simulink model "BatterySOCEstimation_by_me_3"  (R2024b)
settings: Solver=VariableStepAuto  StartTime=0.0  StopTime=1500  FixedStep=Ts  RelTol=1e-3  EnableMultiTasking=on
PreLoadFcn:
  | BatterySOCEstimationData;
libraries: fl_lib x8, nesl_utility x5, simulink x3, batteryecm_lib x1, BatteryEstimators x1
CloseFcn:
  | try
  |     close(h1_BatterySOCEstimation)
  | catch
  | end
  | 
  | clear h1_BatterySOCEstimation
  | 
  | clear BatterySOCEstimationSimlog
  | clear BatterySOCEstimationLogsout
  | 
  | clear AH SOC_vec T_vec R0_mat R1_mat tau1_mat
  | clear V0_mat Q R P0 initialSOC SOC0 Ts
  | clear cell_area h_conv thermal_mass
Description:
  | Battery State-of-Charge Estimation
settings Model: Creator=The MathWorks, Inc.  LastModifiedBy=nikhi
settings SolverCC: AlgebraicLoopSolver=TrustRegion  AutoInsertRateTranBlk=on  MaxZcPerStep=1
settings DataIOCC: MaxDataPoints=370000  ReturnWorkspaceOutputs=off  SignalLoggingName=BatterySOCEstimationLogsout
settings OptimizationCC: ReuseModelBlockBuffer=off  LifeSpan=inf
settings DebuggingCC: UnconnectedInputMsg=warning  UnconnectedOutputMsg=warning  UnconnectedLineMsg=warning  SFUnexpectedBacktrackingDiag=warning  SFNoUnconditionalDefaultTransitionDiag=warning  SFExecutionAtInitializationDiag=none  ArithmeticOperatorsInVariantConditions=warning
settings ModelReferenceCC: EnableRefExpFcnMdlSchedulingChecks=on
settings SFSimCC: SimUseLocalCustomCode=off  CustomCodeUndefinedFunction=UseInterfaceOnly
settings RTWCC: RTWUseLocalCustomCode=off  GPUComputeCapability=3.5  DLArmComputeVersion=19.05
settings CodeAppCC: StateflowObjectComments=on
settings GRTTargetCC: TargetLangStandard=C89/C90 (ANSI)
settings ConfigComp: CovMetricSettings=dw  CovSaveCumulativeToWorkspaceVar=on  CovSaveSingleToWorkspaceVar=on  CovExternalEMLEnable=off
settings SimscapeCC: SimscapeLogType=all  SimscapeLogSimulationStatistics=on  SimscapeLogName=BatterySOCEstimationSimlog  SimscapeLogLimitData=off  SimscapeLogDataHistory=370000

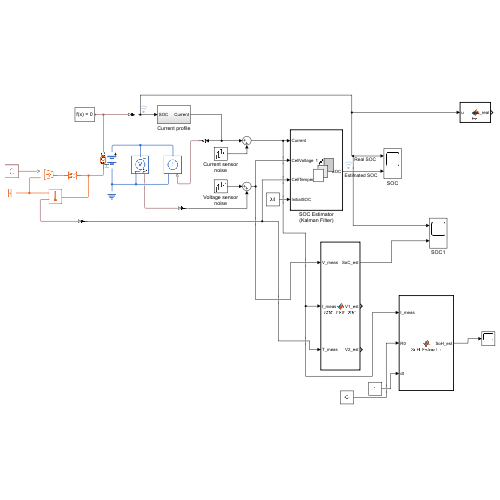
[thumbnail: Simulink's stored preview of the top-level diagram]
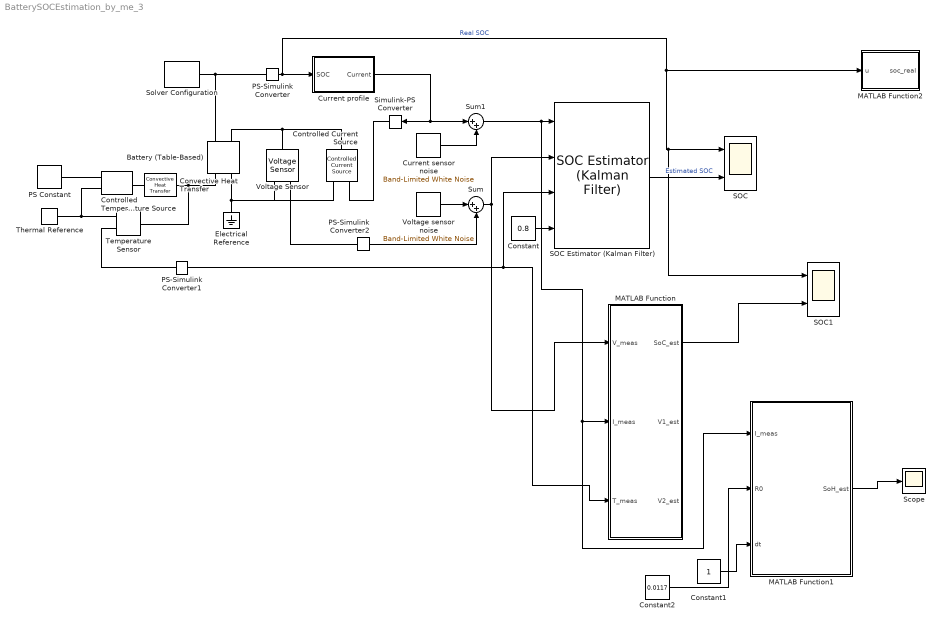
== system BatterySOCEstimation_by_me_3 ==
  Battery (Table-Based) : batteryecm_lib/Battery (Table-Based)  SOC_vec=[0 0.1 0.25 0.5 0.75 0.9 1]  T_dependence=simscape.enum.tablebattery.temperature_dependence.yes  prm_dir=simscape.enum.tablebattery.prm_dir.noCurrentDirectionality  T_vec=[278,293,313] K  V0_mat=[3.49 3.5 3.51;3.55 3.57 3.56;3.62 3.63 3.64;3.71 3.71 3.72;3.91 3.93 3.94;4.07 4.08 4.08;4.19 4.19 4.19] V  V0_vec=[3.5057, 3.566, 3.6337, 3.7127, 3.9259, 4.0777, 4.1928] V  V_range=[0, inf] V  R0_mat=[0.0117 0.0085 0.009;0.011 0.0085 0.009;0.0114 0.0087 0.0092;0.0107 0.0082 0.0088;0.0107 0.0083 0.0091;0.0113 0.0085 0.0089;0.0116 0.0085 0.0089] Ohm  R0_vec=[.0085, .0085, .0087, .0082, .0083, .0085, .0085] Ohm  R0_dis_mat=[.0117, .0085, .009; .011, .0085, .009; .0114, .0087, .0092; .0107, .0082, .0088; .0107, .0083, .0091; .0113, .0085, .0089; .0116, .0085, .0089] Ohm  R0_dis_vec=[.0085, .0085, .0087, .0082, .0083, .0085, .0085] Ohm  R0_ch_mat=[.0117, .0085, .009; .011, .0085, .009; .0114, .0087, .0092; .0107, .0082, .0088; .0107, .0083, .0091; .0113, .0085, .0089; .0116, .0085, .0089] Ohm  R0_ch_vec=[.0085, .0085, .0087, .0082, .0083, .0085, .0085] Ohm  AH=10 A*hr  prm_leak=simscape.enum.tablebattery.prm_leak.disabled  Rleak_vec=[8000, 7000, 6000] Ohm  Rleak=7e3 Ohm  extrapolation_option=simscape.enum.extrapolation.nearest  SOC_port=simscape.enum.tablebattery.enable.yes  prm_dyn=simscape.enum.tablebattery.prm_dyn.rc1  R1_mat=[0.0109 0.0029 0.0013;0.0069 0.0024 0.0012;0.0047 0.0026 0.0013;0.0034 0.0016 0.001;0.0033 0.0023 0.0014;0.0033 0.0018 0.0011;0.0028 0.0017 0.0011] Ohm  R1_vec=[.0029, .0024, .0026, .0016, .0023, .0018, .0017] Ohm  tau1_mat=[20 36 39;31 45 39;109 105 61;36 29 26;59 77 67;40 33 29;25 39 33] s  tau1_vec=[36, 45, 105, 29, 77, 33, 39] s  R2_mat=[.0109, .0029, .0013; .0069, .0024, .0012; .0047, .0026, .0013; .0034, .0016, .001; .0033, .0023, .0014; .0033, .0018, .0011; .0028, .0017, .0011] Ohm  R2_vec=[.0029, .0024, .0026, .0016, .0023, .0018, .0017] Ohm  tau2_mat=[20, 36, 39; 31, 45, 39; 109, 105, 61; 36, 29, 26; 59, 77, 67; 40, 33, 29; 25, 39, 33] s  tau2_vec=[36, 45, 105, 29, 77, 33, 39] s  R3_mat=[.0109, .0029, .0013; .0069, .0024, .0012; .0047, .0026, .0013; .0034, .0016, .001; .0033, .0023, .0014; .0033, .0018, .0011; .0028, .0017, .0011] Ohm  R3_vec=[.0029, .0024, .0026, .0016, .0023, .0018, .0017] Ohm  tau3_mat=[20, 36, 39; 31, 45, 39; 109, 105, 61; 36, 29, 26; 59, 77, 67; 40, 33, 29; 25, 39, 33] s  tau3_vec=[36, 45, 105, 29, 77, 33, 39] s  R4_mat=[.0109, .0029, .0013; .0069, .0024, .0012; .0047, .0026, .0013; .0034, .0016, .001; .0033, .0023, .0014; .0033, .0018, .0011; .0028, .0017, .0011] Ohm  R4_vec=[.0029, .0024, .0026, .0016, .0023, .0018, .0017] Ohm  tau4_mat=[20, 36, 39; 31, 45, 39; 109, 105, 61; 36, 29, 26; 59, 77, 67; 40, 33, 29; 25, 39, 33] s  tau4_vec=[36, 45, 105, 29, 77, 33, 39] s  R5_mat=[.0109, .0029, .0013; .0069, .0024, .0012; .0047, .0026, .0013; .0034, .0016, .001; .0033, .0023, .0014; .0033, .0018, .0011; .0028, .0017, .0011] Ohm  R5_vec=[.0029, .0024, .0026, .0016, .0023, .0018, .0017] Ohm  tau5_mat=[20, 36, 39; 31, 45, 39; 109, 105, 61; 36, 29, 26; 59, 77, 67; 40, 33, 29; 25, 39, 33] s  tau5_vec=[36, 45, 105, 29, 77, 33, 39] s  prm_fade=simscape.enum.tablebattery.prm_fade.disabled  N0=10  dV0=0  dR0=500  dAH=0  dRleak=0  dR1=0  dR2=0  dR3=0  dR4=0  dR5=0  N0vec=[100, 200, 300]  Tfadevec=[298.15, 323.15] K  dV0vec=[0, 0, 0]  dR0vec=[0, 0, 0]  dAHvec=[0, 0, 0]  dRleakvec=[0, 0, 0]  dR1vec=[0, 0, 0]  dR2vec=[0, 0, 0]  dR3vec=[0, 0, 0]  dR4vec=[0, 0, 0]  dR5vec=[0, 0, 0]  dV0mat=[0, 0; 0, 0; 0, 0]  dR0mat=[0, 0; 0, 0; 0, 0]  dAHmat=[0, 0; 0, 0; 0, 0]  dRleakmat=[0, 0; 0, 0; 0, 0]  dR1mat=[0, 0; 0, 0; 0, 0]  dR2mat=[0, 0; 0, 0; 0, 0]  dR3mat=[0, 0; 0, 0; 0, 0]  dR4mat=[0, 0; 0, 0; 0, 0]  dR5mat=[0, 0; 0, 0; 0, 0]  prm_age_modeling=simscape.enum.tablebattery.prm_age_modeling.equation  storage_dt_age_vec=[0] d  storage_T_age_vec=[273] K  prm_age_OCV=simscape.enum.tablebattery.prm_age_OCV.OCV  OCV_age=0.9  SOC_age=0.6  prm_age_resistance=simscape.enum.tablebattery.prm_age.disabled  OCV_scaling_age_resistance=2.2134e6  OCV_offset_age_resistance=1.632e6  temp_exp_age_resistance=0.515833569 V  t_exp_age_resistance=0.75  T_age_vec_resistance=[273.15, 298.15, 323.15] K  dt_age_vec_resistance=[90, 180, 270, 360] d  dR0_age_vec=[0, 0, 0]  t_meas_dR0_age=100 d  dR0_age_mat=[0, 0, 0; 0, 0, 0; 0, 0, 0; 0, 0, 0]  prm_age_capacity=simscape.enum.tablebattery.prm_age.disabled  OCV_scaling_age_capacity=1.5097e07  OCV_offset_age_capacity=8.3625e06  temp_exp_age_capacity=0.6011 V  t_exp_age_capacity=0.75  T_age_vec_capacity=[273.15, 298.15, 323.15] K  dt_age_vec_capacity=[90, 180, 270, 360] d  dAH_age_vec=[0, 0, 0]  t_meas_dAH_age=100 d  dAH_age_mat=[0, 0, 0; 0, 0, 0; 0, 0, 0; 0, 0, 0]  thermal_port=simscape.enum.thermaleffects.model  temperature=298.15 K  thermal_mass=100 J/K  i_specify=off  i_priority=None  i=0 A  i_nominal_specify=off  i_nominal_value=1  i_nominal_unit=A  v_specify=off  v_priority=None  v=0 V  v_nominal_specify=off  v_nominal_value=1  v_nominal_unit=V  stateOfCharge_specify=on  stateOfCharge_priority=High  stateOfCharge=0.5  stateOfCharge_nominal_specify=off  stateOfCharge_nominal_value=1  stateOfCharge_nominal_unit=1  num_cycles_specify=off  num_cycles_priority=High  num_cycles=0  num_cycles_nominal_specify=off  num_cycles_nominal_value=1  num_cycles_nominal_unit=1  cell_temperature_specify=off  cell_temperature_priority=High  cell_temperature=293.15 K  cell_temperature_nominal_specify=off  cell_temperature_nominal_value=1  cell_temperature_nominal_unit=K
  Constant : Constant  Value=0.8
  Constant1 : Constant
  Constant2 : Constant  Value=0.0117
  Controlled Temperature Source : fl_lib/Thermal/Thermal Sources/Controlled Temperature Source
  Controlled Current Source : fl_lib/Electrical/Electrical Sources/Controlled Current Source
  Convective Heat Transfer : fl_lib/Thermal/Thermal Elements/Convective Heat Transfer  thermal_type=foundation.enum.constant_variable.constant  area=0.1019 m^2  heat_tr_coeff=5 W/(K*m^2)  min_heat_tr_coeff=1e-3 W/(K*m^2)  T_specify=off  T_priority=None  T=0 K  T_nominal_specify=off  T_nominal_value=1  T_nominal_unit=K  Q_specify=off  Q_priority=None  Q=0 W  Q_nominal_specify=off  Q_nominal_value=1  Q_nominal_unit=W
  Current profile : Subsystem
  Current sensor noise : simulink/Sources/Band-Limited White Noise  Cov=1e-2  Ts=1  seed=1234
  Electrical Reference : fl_lib/Electrical/Electrical Elements/Electrical Reference
  MATLAB Function : MATLAB Function  TreatAsAtomicUnit=on
  MATLAB Function1 : MATLAB Function  TreatAsAtomicUnit=on
  MATLAB Function2 : MATLAB Function  TreatAsAtomicUnit=on
  PS Constant : fl_lib/Physical Signals/Sources/PS Constant  constant=292.15 K
  PS-Simulink Converter : nesl_utility/PS-Simulink Converter  PhysicalDomain=network_engine_domain  SubClassName=ps_output  LeftPortType=input  RightPortType=output  PseudoPeriodic=off  Frequencies=[]  VectorFormat=inherit  Unit=inherit  AffineConversion=off
  PS-Simulink Converter1 : nesl_utility/PS-Simulink Converter  PhysicalDomain=network_engine_domain  SubClassName=ps_output  LeftPortType=input  RightPortType=output  PseudoPeriodic=off  Frequencies=[]  VectorFormat=inherit  Unit=inherit  AffineConversion=off
  PS-Simulink Converter2 : nesl_utility/PS-Simulink Converter  PhysicalDomain=network_engine_domain  SubClassName=ps_output  LeftPortType=input  RightPortType=output  PseudoPeriodic=off  Frequencies=[]  VectorFormat=inherit  Unit=inherit  AffineConversion=off
  SOC : Scope  NumInputPorts=2
  SOC Estimator (Kalman Filter) : BatteryEstimators/SOC Estimator (Kalman Filter)  CurrentInputPartition=off  filterType=Extended Kalman filter  alpha=1  beta=2  kappa=0  Q=[0.0001,0;0,0.0001]  Q_2RC=|  R=0.7  P0=[1e-05,0;0,1]  P0_2RC=[1e-5 0 0; 0 1 0;0 0 1]  Ts=1  chargeDynamics=One time-constant dynamics  SOC_vec=[0 0.1 0.25 0.5 0.75 0.9 1]  T_vec=[278,293,313]  R0_mat=[0.0117 0.0085 0.009;0.011 0.0085 0.009;0.0114 0.0087 0.0092;0.0107 0.0082 0.0088;0.0107 0.0083 0.0091;0.0113 0.0085 0.0089;0.0116 0.0085 0.0089]  R1_mat=[0.0109 0.0029 0.0013;0.0069 0.0024 0.0012;0.0047 0.0026 0.0013;0.0034 0.0016 0.001;0.0033 0.0023 0.0014;0.0033 0.0018 0.0011;0.0028 0.0017 0.0011]  tau1_mat=[20 36 39;31 45 39;109 105 61;36 29 26;59 77 67;40 33 29;25 39 33]  R2_mat=[.0109, .0029, .0013; .0069, .0024, .0012; .0047, .0026, .0013; .0034, .0016, .001; .0033, .0023, .0014; .0033, .0018, .0011; .0028, .0017, .0011]  tau2_mat=[20, 36, 39; 31, 45, 39; 109, 105, 61; 36, 29, 26; 59, 77, 67; 40, 33, 29; 25, 39, 33]  V0_mat=[3.49 3.5 3.51;3.55 3.57 3.56;3.62 3.63 3.64;3.71 3.71 3.72;3.91 3.93 3.94;4.07 4.08 4.08;4.19 4.19 4.19]  AH=10
      | [1e-6 0 0;
      | 0 1e-6 0; 0 0 1e-6]
  SOC1 : Scope  NumInputPorts=2
  Scope : Scope
  Simulink-PS Converter : nesl_utility/Simulink-PS Converter  PhysicalDomain=network_engine_domain  SubClassName=ps_input  LeftPortType=input  RightPortType=output  PseudoPeriodic=off  Frequencies=[]  NoiseDistribution=none  NoiseParameters=[]  Unit=1  AffineConversion=off  FilteringAndDerivatives=provide  SimscapeFilterOrder=1  InputFilterTimeConstant=0.001  UdotUserProvided=0
  Solver Configuration : nesl_utility/Solver Configuration  PhysicalDomain=network_engine_domain  SubClassName=solver  LeftPortType=input  RightPortType=generic  Tones=[]  Harmonics=[]  SimulateNoise=off  Profile=off  UseLocalSampling=off  EnableSwitchedLinearOptims=on  FrequencyDomain=off  UseCCode=off  RelTol=0.001  AbsTol=0.001  MinStep=1e-09  ToWorkspace=off  RevertToSquareIcSolve=off  NumHomotopyIterations=100  PhasorMode=off  PhasorModeNumHarmonics=1  ConsistencySolver=NEWTON_XTOL_AFTER_FTOL  IndexReductionMethod=DerivativeReplacement  DoDC=off  ResidualTolerance=1e-09  ConsistencyTolSource=GLOBAL  ConsistencyAbsTol=0.001  ConsistencyRelTol=0.001  ConsistencyTolFactor=0.001  UseLocalSolver=on  LocalSolverChoice=NE_BACKWARD_EULER_ADVANCER  ResolveIndetEquations=on  FunctionEvalNumThread=1  LocalSolverSampleTime=1  DoFixedCost=on  MaxNonlinIter=3  MaxModeIter=2  ComputeImpulses=off  ImpulseIterations=2  LinearAlgebra=auto  LinearAlgebraNumThread=0  EquationFormulation=NE_TIME_EF  DelaysMemoryBudget=1024  AutomaticFiltering=on  FilteringTimeConstant=0.001  PartitionStorageMethod=AS_NEEDED  PartitionMemoryBudget=1024  PartitionMethod=ROBUST  MultibodyUseLocalSolver=off  MultibodyLocalSolverChoice=ODE1  MultibodyLocalSolverSampleTime=0.001
  Sum : Sum  Inputs=|++
  Sum1 : Sum  Inputs=|++
  Temperature Sensor : fl_lib/Thermal/Thermal Sensors/Temperature Sensor  temperature_measure=foundation.enum.MeasurementReference.difference
  Thermal Reference : fl_lib/Thermal/Thermal Elements/Thermal Reference
  Voltage Sensor : fl_lib/Electrical/Electrical Sensors/Voltage Sensor
  Voltage sensor noise : simulink/Sources/Band-Limited White Noise  Cov=1e-2  Ts=1  seed=1234
  wires:
  PS-Simulink Converter2/1 -> Sum/2
  Current sensor noise/1 -> Sum1/2
  Constant/1 -> SOC Estimator (Kalman Filter)/4
  SOC Estimator (Kalman Filter)/1 -> SOC/2  "Estimated SOC"
  PS-Simulink Converter/1 -> MATLAB Function2/1(u), SOC1/1, SOC/1, Current profile/1(SOC)  "Real SOC"
  Voltage sensor noise/1 -> Sum/1
  Current profile/1(Current) -> Sum1/1, Simulink-PS Converter/1
  MATLAB Function/1(SoC_est) -> SOC1/2
  Sum/1 -> MATLAB Function/1(V_meas), SOC Estimator (Kalman Filter)/2
  Sum1/1 -> MATLAB Function1/1(I_meas), MATLAB Function/2(I_meas), SOC Estimator (Kalman Filter)/1
  PS-Simulink Converter1/1 -> MATLAB Function/3(T_meas), SOC Estimator (Kalman Filter)/3
  Constant1/1 -> MATLAB Function1/3(dt)
  Constant2/1 -> MATLAB Function1/2(R0)
  MATLAB Function1/1(SoH_est) -> Scope/1
  connections:
  PS-Simulink Converter/LConn1 -- Solver Configuration/RConn1 -- Battery (Table-Based)/LConn2
  Convective Heat Transfer/LConn1 -- Temperature Sensor/LConn1 -- Battery (Table-Based)/RConn2
  Controlled Temperature Source/LConn1 -- Convective Heat Transfer/RConn1
  Thermal Reference/LConn1 -- Controlled Temperature Source/RConn2 -- Temperature Sensor/RConn1
  PS-Simulink Converter1/LConn1 -- Temperature Sensor/RConn2
  Electrical Reference/LConn1 -- Voltage Sensor/RConn2 -- Controlled Current Source/RConn2 -- Battery (Table-Based)/RConn1
  Voltage Sensor/LConn1 -- Controlled Current Source/LConn1 -- Battery (Table-Based)/LConn1
  Simulink-PS Converter/RConn1 -- Controlled Current Source/RConn1
  Voltage Sensor/RConn1 -- PS-Simulink Converter2/LConn1
  PS Constant/RConn1 -- Controlled Temperature Source/RConn1

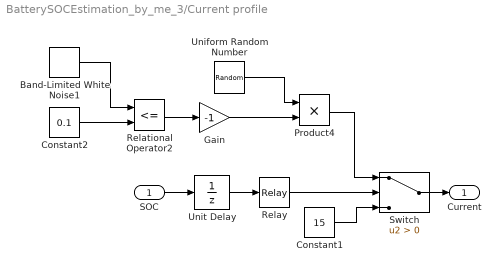
== system BatterySOCEstimation_by_me_3/Current profile ==
  SOC : Inport
  Band-Limited White Noise1 : simulink/Sources/Band-Limited White Noise  Cov=1  Ts=50  seed=[23341]
  Constant1 : Constant  Value=15
  Constant2 : Constant  Value=0.1
  Gain : Gain  Gain=-1
  Product4 : Product
  Relational Operator2 : RelationalOperator  Operator=<=  OutDataTypeStr=boolean  RndMeth=Simplest  InputSameDT=off
  Relay : Relay  OnSwitchValue=0.9  OffSwitchValue=0.3  OffOutputValue=-1
  Switch : Switch  Criteria=u2 > Threshold  SaturateOnIntegerOverflow=off  InputSameDT=off
  Uniform Random Number : UniformRandomNumber  Minimum=5  Maximum=55  SampleTime=100
  Unit Delay : UnitDelay  HasFrameUpgradeWarning=on
  Current : Outport
  wires:
  SOC/1 -> Unit Delay/1
  Constant1/1 -> Switch/3
  Relay/1 -> Switch/2
  Product4/1 -> Switch/1
  Unit Delay/1 -> Relay/1
  Switch/1 -> Current/1
  Uniform Random Number/1 -> Product4/1
  Band-Limited White Noise1/1 -> Relational Operator2/1
  Gain/1 -> Product4/2
  Relational Operator2/1 -> Gain/1
  Constant2/1 -> Relational Operator2/2

== matlab function BatterySOCEstimation_by_me_3/MATLAB Function1 ==
  data: I_meas input; SoH_est output; R0 input; dt input
function SoH_est = SoH_Estimator(I_meas, R0, dt)
% SoH_Estimator - Estimates battery State of Health (SoH)
%
% Inputs:
%   I_meas : Measured battery current [A] (+ve discharge, -ve charge)
%   R0     : Instantaneous internal resistance [Ohm]
%   dt     : Sample time [s]
%
% Output:
%   SoH_est : Estimated state of health (0-1)

%% Persistent variables to track battery history
persistent Q_used C_est R0_ref C_rated

if isempty(R0_ref)
    Q_used  = 0;          % cumulative charge throughput [Ah]
    C_rated = 2.3;        % rated capacity in Ah (modify for your battery)
    C_est   = C_rated;    % initialize capacity estimate
    R0_ref  = mean(R0);   % reference R0 for fresh battery
end

%% --- Update cumulative charge throughput
Q_used = Q_used + abs(I_meas) * dt / 3600;  % convert A*s to Ah

%% --- Capacity fade model (adaptive)
alpha_cap = 1e-5;  % slow adaptation factor
C_est = (1 - alpha_cap)*C_est + alpha_cap*(C_rated - Q_used);

%% --- Resistance-based SoH
SoH_res = R0_ref ./ R0;

%% --- Capacity-based SoH
SoH_cap = C_est / C_rated;

%% --- Combine SoH estimates (average)
SoH_est = 0.5*(SoH_res + SoH_cap);

%% --- Optional: Clip SoH between 0 and 1
SoH_est = max(0, min(1, SoH_est));

end

== matlab function BatterySOCEstimation_by_me_3/MATLAB Function ==
  data: V_meas input; I_meas input; SoC_est output; T_meas input; V1_est output; V2_est output
function [SoC_est, V1_est, V2_est] = SOC_EKF_2RC(V_meas, I_meas, T_meas)
persistent x P dt Q R soc_grid temp_grid R0_data R1_data R2_data tau1_data tau2_data V0_data Cbat

if isempty(x)
    dt = 1; % sample time in seconds
    Cbat = 2.3; % battery nominal capacity [Ah], change as per your battery

    % Initial state [SOC; V1; V2]
    x = double([0.8; 0; 0]);

    % Initial error covariance
    P = double(diag([1e-4, 1e-3, 1e-3]));

    % Process noise covariance
    Q = double(diag([1e-4, 1e-4, 1e-4]));

    % Measurement noise covariance
    R = double(0.7^2);

    % SOC and temperature grids
    soc_grid = double([0 0.1 0.25 0.5 0.75 0.9 1]);
    temp_grid = double([278 293 313]);

    % Battery parameters tables (example matrices)
    R0_data = double([0.0117 0.0085 0.009;
                      0.011 0.0085 0.009;
                      0.0114 0.0087 0.0092;
                      0.0107 0.0082 0.0088;
                      0.0107 0.0083 0.0091;
                      0.0113 0.0085 0.0089;
                      0.0116 0.0085 0.0089]);

    R1_data = double([0.0109 0.0029 0.0013;
                      0.0069 0.0024 0.0012;
                      0.0047 0.0026 0.0013;
                      0.0034 0.0016 0.001;
                      0.0033 0.0023 0.0014;
                      0.0033 0.0018 0.0011;
                      0.0028 0.0017 0.0011]);

    R2_data = double([0.003 0.002 0.0015;
                      0.0025 0.0018 0.0012;
                      0.002 0.0015 0.001;
                      0.0018 0.0013 0.0009;
                      0.0016 0.0012 0.0008;
                      0.0015 0.001 0.0007;
                      0.0014 0.0009 0.0006]);

    tau1_data = double([20 36 39;
                        31 45 39;
                        109 105 61;
                        36 29 26;
                        59 77 67;
                        40 33 29;
                        25 39 33]);

    tau2_data = double([200 180 150;
                        220 200 170;
                        300 280 250;
                        180 160 140;
                        250 230 210;
                        200 180 150;
                        150 140 130]);

    V0_data = double([3.49 3.5 3.51;
                      3.55 3.57 3.56;
                      3.62 3.63 3.64;
                      3.71 3.71 3.72;
                      3.91 3.93 3.94;
                      4.07 4.08 4.08;
                      4.19 4.19 4.19]);
end

% Clamp inputs
T_meas = max(min(T_meas, temp_grid(end)), temp_grid(1));
SoC_clamped = max(min(x(1), soc_grid(end)), soc_grid(1));

% Interpolate parameters
R0 = interp2(temp_grid, soc_grid, R0_data, T_meas, SoC_clamped,'linear');
R1 = interp2(temp_grid, soc_grid, R1_data, T_meas, SoC_clamped,'linear');
R2 = interp2(temp_grid, soc_grid, R2_data, T_meas, SoC_clamped,'linear');
tau1 = interp2(temp_grid, soc_grid, tau1_data, T_meas, SoC_clamped,'linear');
tau2 = interp2(temp_grid, soc_grid, tau2_data, T_meas, SoC_clamped,'linear');
V0 = interp2(temp_grid, soc_grid, V0_data, T_meas, SoC_clamped,'linear');

% Clamp interpolated values
R0 = max(min(R0,max(R0_data(:))),min(R0_data(:)));
R1 = max(min(R1,max(R1_data(:))),min(R1_data(:)));
R2 = max(min(R2,max(R2_data(:))),min(R2_data(:)));
tau1 = max(min(tau1,max(tau1_data(:))),min(tau1_data(:)));
tau2 = max(min(tau2,max(tau2_data(:))),min(tau2_data(:)));
V0 = max(min(V0,max(V0_data(:))),min(V0_data(:)));

% Compute capacitances
C1 = tau1/R1;
C2 = tau2/R2;

%% Prediction step
x_pred = zeros(3,1,'double');
x_pred(1) = x(1) - dt*I_meas/(Cbat*3600);
x_pred(2) = x(2) + dt*(-x(2)/(R1*C1) + I_meas/C1);
x_pred(3) = x(3) + dt*(-x(3)/(R2*C2) + I_meas/C2);

% Jacobian
F = double([1 0 0;
            0 1-dt/(R1*C1) 0;
            0 0 1-dt/(R2*C2)]);
P_pred = F*P*F' + Q;

%% Measurement update
V_est = V0 - x_pred(2) - x_pred(3) - I_meas*R0;

% SOC slope (dV0/dSOC)
dV0_dSOC = gradient(V0_data(:,1), soc_grid); % approximate slope
dV0dSOC_interp = interp1(soc_grid,dV0_dSOC,SoC_clamped,'linear','extrap');

H = [dV0dSOC_interp -1 -1];
y = V_meas - V_est;
S = H*P_pred*H' + R;
K = P_pred*H'/S;

x = x_pred + K*y;
P = (eye(3,'double') - K*H)*P_pred;

% Outputs
SoC_est = x(1);
V1_est = x(2);
V2_est = x(3);
end

== matlab function BatterySOCEstimation_by_me_3/MATLAB Function2 ==
  data: u input; soc_real output
function soc_real = fcn(u)

soc_real = u
